simulink model "questao7_talvezsejaesseocaminho"  (R2022b)
settings: Solver=VariableStepAuto  StartTime=0.0  StopTime=15  RelTol=1e-3
settings Model: Creator=13199959938  LastModifiedBy=maria
settings SolverCC: AlgebraicLoopSolver=TrustRegion
settings DataIOCC: ReturnWorkspaceOutputs=off
settings DebuggingCC: UnconnectedInputMsg=warning  UnconnectedOutputMsg=warning  UnconnectedLineMsg=warning  SFMachineParentedDataDiag=warning  ArithmeticOperatorsInVariantConditions=warning
settings ModelReferenceCC: EnableRefExpFcnMdlSchedulingChecks=on
settings SFSimCC: SimUseLocalCustomCode=off  CustomCodeUndefinedFunction=UseInterfaceOnly
settings RTWCC: RTWUseLocalCustomCode=off
settings CodeAppCC: StateflowObjectComments=on

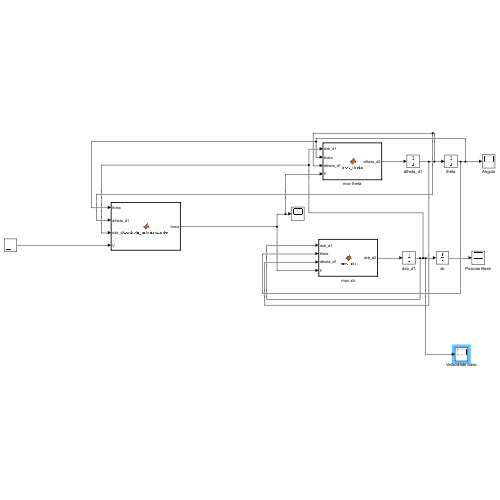
[thumbnail: Simulink's stored preview of the top-level diagram]
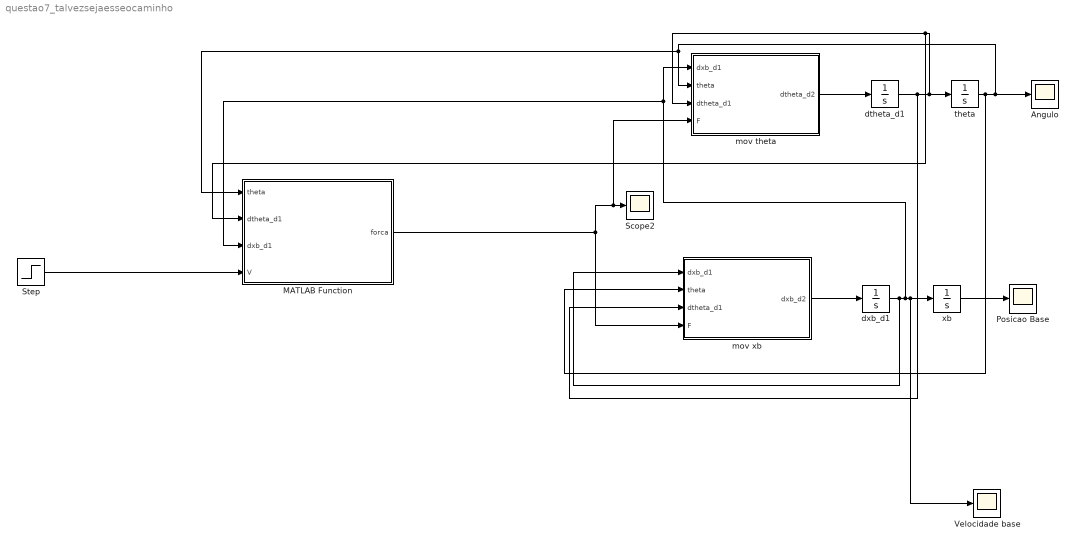
== system questao7_talvezsejaesseocaminho ==
  Angulo : Scope
  MATLAB Function : MATLAB Function  TreatAsAtomicUnit=on
  Posicao Base : Scope
  Scope2 : Scope
  Step : Step  After=5  SampleTime=0
  Velocidade base : Scope
  dtheta_d1 : Integrator
  dxb_d1 : Integrator
  mov theta : MATLAB Function  TreatAsAtomicUnit=on
  mov xb : MATLAB Function  TreatAsAtomicUnit=on
  theta : Integrator
  xb : Integrator
  wires:
  mov xb/1(dxb_d2) -> dxb_d1/1
  mov theta/1(dtheta_d2) -> dtheta_d1/1
  dtheta_d1/1 -> mov xb/3(dtheta_d1), MATLAB Function/2(dtheta_d1), mov theta/3(dtheta_d1), theta/1
  theta/1 -> mov xb/2(theta), mov theta/2(theta), MATLAB Function/1(theta), Angulo/1
  dxb_d1/1 -> mov xb/1(dxb_d1), mov theta/1(dxb_d1), MATLAB Function/3(dxb_d1), Velocidade base/1, xb/1
  xb/1 -> Posicao Base/1
  MATLAB Function/1(forca) -> mov theta/4(F), Scope2/1, mov xb/4(F)
  Step/1 -> MATLAB Function/4(V)

== matlab function questao7_talvezsejaesseocaminho/mov xb ==
  data: dxb_d1 input; dxb_d2 output; theta input; dtheta_d1 input; F input
function dxb_d2 = mov_xb(dxb_d1, theta, dtheta_d1, F)
    g = 9.81; % m/s^2
    l = 1.30; % m
    m = 120; % kg
    M = 54; % kg
    b = 250; % atrito viscoso com o ar
    d = 97.2; % Ns/M
    
    dxb_d2 = (F-d*dxb_d1-m*l*sin(theta)*dtheta_d1^2+m*g*sin(theta)*cos(theta)-(b*dtheta_d1*cos(theta))/l)/((M+m*(sin(theta))^2));

== matlab function questao7_talvezsejaesseocaminho/mov theta ==
  data: dxb_d1 input; dtheta_d2 output; theta input; dtheta_d1 input; F input
function dtheta_d2 = mov_theta(dxb_d1, theta, dtheta_d1, F)
    g = 9.81; % m/s^2
    l = 1.30; % m
    m = 120; % kg
    M = 54; % kg
    b = 250; % atrito viscoso com o ar
    d = 97.2; % Ns/M
    
    dtheta_d2 = ((M+m)*g*l*sin(theta)+l*cos(theta)*(F-d*dxb_d1-m*l*sin(theta)*dtheta_d1^2)-((M+m)*b*dtheta_d1)/m)/(l^2*(M+m*(sin(theta))^2));

== matlab function questao7_talvezsejaesseocaminho/MATLAB Function ==
  data: theta input; forca output; dtheta_d1 input; dxb_d1 input; V input
function forca = controle_relinearizante(theta, dtheta_d1, dxb_d1, V)
    g = 9.81; % m/s^2
    l = 1.30; % m
    m = 120; % kg
    M = 54; % kg
    b = 1.3; % atrito viscoso com o ar
    d = 97.2; % Ns/M

    forca = (-(M+m)*l*g*sin(theta) +m*l^2*sin(theta)*cos(theta)*dtheta_d1^2 + d*l*cos(theta)*dxb_d1+V) / (l*cos(theta));
